simulink model "gm_test_cost_function_only_without_delays"  (R2022a)
settings: Solver=FixedStepDiscrete  StartTime=0.0  StopTime=10.0  RelTol=1e-3
undefined symbols (not defined in the file or in its folder): f_c
libraries: hdlmdlgenlib x64
(part 1 of 2)
settings Model: Creator=Andre Merx  LastModifiedBy=Andre Merx
settings SolverCC: AlgebraicLoopSolver=TrustRegion
settings DataIOCC: LimitDataPoints=on  SaveOutput=off  SaveTime=off
settings OptimizationCC: BlockReduction=off  ConditionallyExecuteInputs=off  DefaultParameterBehavior=Inlined  LifeSpan=inf
settings DebuggingCC: AlgebraicLoopMsg=error  InheritedTsInSrcMsg=none  SingleTaskRateTransMsg=error  UnconnectedInputMsg=warning  UnconnectedOutputMsg=warning  UnconnectedLineMsg=warning  AllowSymbolicDim=off  StrictBusMsg=ErrorOnBusTreatedAsVector  SFUnexpectedBacktrackingDiag=warning  SFNoUnconditionalDefaultTransitionDiag=warning  SFExecutionAtInitializationDiag=none  SFMachineParentedDataDiag=warning  ArithmeticOperatorsInVariantConditions=warning
settings HardwareCC: ProdBitPerPointer=32  ProdBitPerSizeT=32  ProdBitPerPtrDiffT=32  ProdLargestAtomicFloat=None  ProdIntDivRoundTo=Undefined  ProdEndianess=Unspecified  ProdWordSize=32  ProdHWDeviceType=ASIC/FPGA->ASIC/FPGA  ProdEqTarget=off
settings SFSimCC: SimUseLocalCustomCode=off  CustomCodeUndefinedFunction=UseInterfaceOnly
settings RTWCC: RTWUseLocalCustomCode=off
settings CodeAppCC: StateflowObjectComments=on
settings GRTTargetCC: TargetLangStandard=C89/C90 (ANSI)
settings ConfigComp: CovScope=ReferencedModels  CovMetricSettings=dw  CovSaveCumulativeToWorkspaceVar=on  CovSaveSingleToWorkspaceVar=on  CovExternalEMLEnable=off  CovSFcnEnable=off

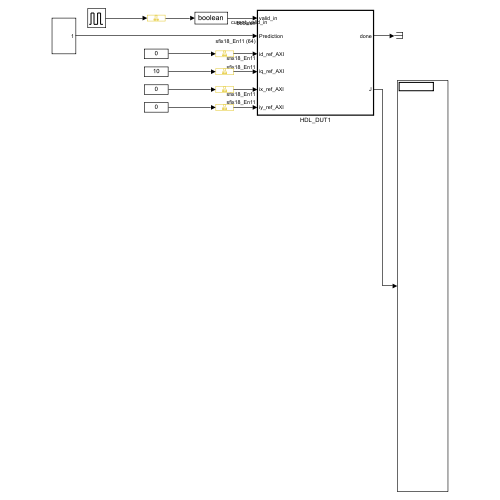
[thumbnail: Simulink's stored preview of the top-level diagram]
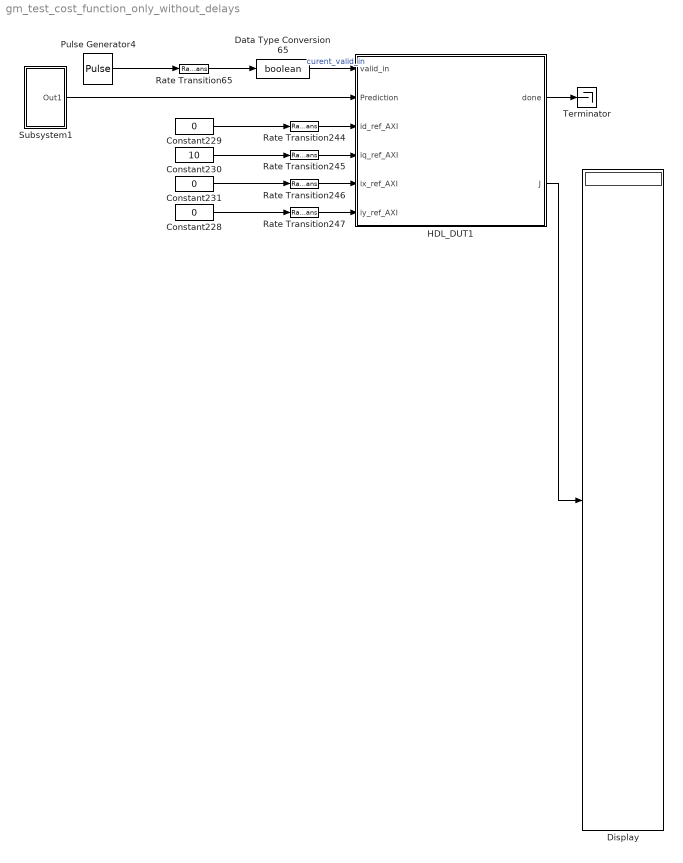
== system gm_test_cost_function_only_without_delays ==
  Constant228 : Constant  Value=0  OutDataTypeStr=fixdt(1,18,11)  SampleTime=-1
  Constant229 : Constant  Value=0  OutDataTypeStr=fixdt(1,18,11)  SampleTime=-1
  Constant230 : Constant  Value=10  OutDataTypeStr=fixdt(1,18,11)  SampleTime=-1
  Constant231 : Constant  Value=0  OutDataTypeStr=fixdt(1,18,11)  SampleTime=-1
  Data Type Conversion65 : DataTypeConversion  OutDataTypeStr=boolean  SaturateOnIntegerOverflow=off  RndMeth=Floor
  Display : Display
  HDL_DUT1 : Subsystem  TreatAsAtomicUnit=on
  Pulse Generator4 : DiscretePulseGenerator  PulseType=Time based  Period=1/f_c
  Rate Transition{65,244..247} (5 alike) : RateTransition  OutPortSampleTime=Rt
  Subsystem1 : Subsystem
  Terminator : Terminator
  wires:
  HDL_DUT1/2(J) -> Display/1
  HDL_DUT1/1(done) -> Terminator/1
  Data Type Conversion65/1 -> HDL_DUT1/1(valid_in)  "curent_valid_in"
  Rate Transition65/1 -> Data Type Conversion65/1
  Pulse Generator4/1 -> Rate Transition65/1
  Rate Transition244/1 -> HDL_DUT1/3(id_ref_AXI)
  Rate Transition246/1 -> HDL_DUT1/5(ix_ref_AXI)
  Constant230/1 -> Rate Transition245/1
  Constant229/1 -> Rate Transition244/1
  Subsystem1/1(Out1) -> HDL_DUT1/2(Prediction)
  Rate Transition245/1 -> HDL_DUT1/4(iq_ref_AXI)
  Rate Transition247/1 -> HDL_DUT1/6(iy_ref_AXI)
  Constant231/1 -> Rate Transition246/1
  Constant228/1 -> Rate Transition247/1

== system gm_test_cost_function_only_without_delays/HDL_DUT1 ==
  valid_in : Inport  OutDataTypeStr=boolean  PortDimensions=1  SampleTime=1e-08
  Prediction : Inport  Port=2  OutDataTypeStr=fixdt(1, 18, 11)  PortDimensions=[64]  SampleTime=1e-08
  id_ref_AXI : Inport  Port=3  OutDataTypeStr=fixdt(1, 18, 11)  PortDimensions=1  SampleTime=1e-08
  iq_ref_AXI : Inport  Port=4  OutDataTypeStr=fixdt(1, 18, 11)  PortDimensions=1  SampleTime=1e-08
  ix_ref_AXI : Inport  Port=5  OutDataTypeStr=fixdt(1, 18, 11)  PortDimensions=1  SampleTime=1e-08
  iy_ref_AXI : Inport  Port=6  OutDataTypeStr=fixdt(1, 18, 11)  PortDimensions=1  SampleTime=1e-08
  Delay{7..10,33} (5 alike) : Delay  DelayLength=double(1)  InitialCondition=0  SampleTime=1e-08
  Detect Rise Positive : Subsystem  mask(Detect Rise Positive){vinit=double(0), InputProcessing=Elements as channels (sample based), OutDataTypeStr=boolean}
      mask prompts: vinit "Simulink:masks:InitialCondition_MP"; InputProcessing "Simulink:masks:InputProcessing_MP"; OutDataTypeStr "Simulink:masks:OutputDataType_MP"
      mask help: Simulink:masks:DetectRisePositive_MD
      mask init:
      | InputProcessing = 'Elements as channels (sample based)';
      | OutDataTypeStr = 'boolean';
      | vinit = double(0);
      mask TypeOptions InputProcessing: Simulink:masks:ColumnsAsChannelsFrameBased | Simulink:masks:ElementsAsChannelsSampleBased
      mask TypeOptions OutDataTypeStr: Simulink:masks:uint8 | Simulink:masks:boolean
      mask Display: fprintf('U > 0\n&  NOT\nU/z > 0')
  Subsystem : Subsystem
  Switch_on{1..4,14} (5 alike) : Switch  Threshold=double(1)  OutDataTypeStr=fixdt(1, 18, 11)  RndMeth=Simplest  SampleTime=1e-08  SaturateOnIntegerOverflow=off  InputSameDT=off
  mux : Mux  Inputs=16
  done : Outport  SampleTime=1e-08
  J : Outport  Port=2  SampleTime=1e-08
  wires:
  valid_in/1 -> Detect Rise Positive/1(U)
  Prediction/1 -> Switch_on4/1
  id_ref_AXI/1 -> Switch_on3/1
  iq_ref_AXI/1 -> Switch_on2/1
  ix_ref_AXI/1 -> Switch_on1/1
  iy_ref_AXI/1 -> Switch_on14/1
  Delay10/1 -> Switch_on4/3
  Delay33/1 -> Switch_on14/3
  Delay7/1 -> Switch_on1/3
  Delay8/1 -> Switch_on2/3
  Delay9/1 -> Switch_on3/3
  Detect Rise Positive/1(Y) -> Switch_on4/2, Switch_on3/2, Switch_on2/2, Switch_on14/2, Switch_on1/2, done/1
  mux/1 -> J/1
  Subsystem/1(J1) -> mux/1
  Subsystem/2(J2) -> mux/2
  Subsystem/3(J3) -> mux/3
  Subsystem/4(J4) -> mux/4
  Subsystem/5(J5) -> mux/5
  Subsystem/6(J6) -> mux/6
  Subsystem/7(J7) -> mux/7
  Subsystem/8(J8) -> mux/8
  Subsystem/9(J9) -> mux/9
  Subsystem/10(J10) -> mux/10
  Subsystem/11(J11) -> mux/11
  Subsystem/12(J12) -> mux/12
  Subsystem/13(J13) -> mux/13
  Subsystem/14(J14) -> mux/14
  Subsystem/15(J15) -> mux/15
  Subsystem/16(J16) -> mux/16
  Switch_on1/1 -> Delay7/1, Subsystem/4(ix_ref)
  Switch_on14/1 -> Delay33/1, Subsystem/5(iy_ref)
  Switch_on2/1 -> Delay8/1, Subsystem/3(iq_ref)
  Switch_on3/1 -> Delay9/1, Subsystem/2(id_ref)
  Switch_on4/1 -> Delay10/1, Subsystem/1(Predicton)

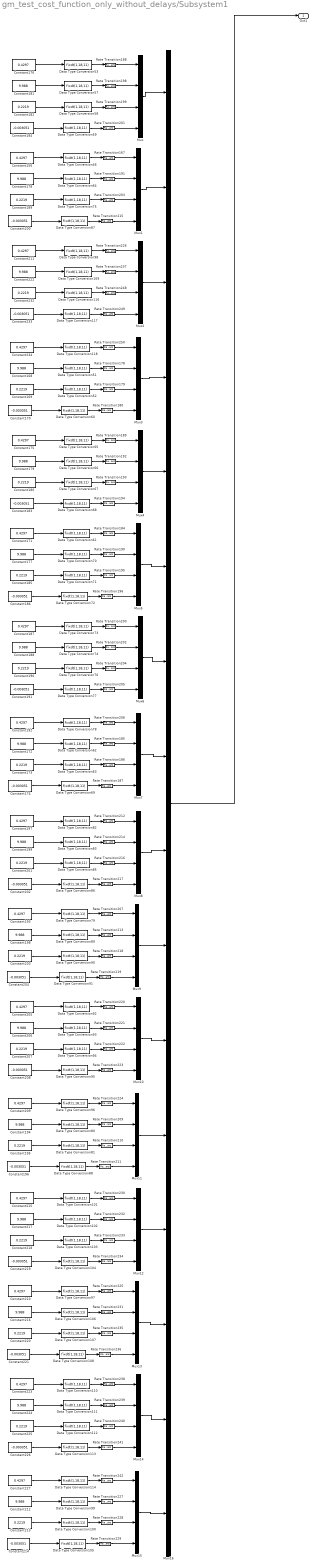
== system gm_test_cost_function_only_without_delays/Subsystem1 ==
  Constant{156,171,175..176,187,192..193,197,205,209..211,215,223,227,234} (16 alike) : Constant  Value=0.4297
  Constant{168,172,177..179,181,188,194,198..199,206,212,216..217,222,224} (16 alike) : Constant  Value=9.988
  Constant{169,173,180,182,185,189..190,195,201,203,207,213,218,220,225,232} (16 alike) : Constant  Value=0.2219
  Constant{170,174,183..184,186,191,196,200,202,204,208,214,219,221,226,233} (16 alike) : Constant  Value=-0.003051
  Data Type Conversion{46,51..53,57..83,85..114,116..118} (64 alike) : DataTypeConversion  OutDataTypeStr=fixdt(1,18,11)  SaturateOnIntegerOverflow=off  RndMeth=Floor
  Mux{,1..15} (16 alike) : Mux
  Mux16 : Mux  Inputs=16
  Rate Transition{167,178..180,184..196,198..207,209..242,248..250} (64 alike) : RateTransition  OutPortSampleTime=Rt
  Out1 : Outport
  wires:
  Data Type Conversion90/1 -> Rate Transition218/1
  Rate Transition223/1 -> Mux10/4
  Data Type Conversion92/1 -> Rate Transition220/1
  Constant197/1 -> Data Type Conversion82/1
  Rate Transition214/1 -> Mux8/2
  Rate Transition206/1 -> Mux7/1
  Data Type Conversion95/1 -> Rate Transition223/1
  Constant207/1 -> Data Type Conversion94/1
  Rate Transition221/1 -> Mux10/2
  Data Type Conversion51/1 -> Rate Transition178/1
  Data Type Conversion89/1 -> Rate Transition213/1
  Rate Transition185/1 -> Mux7/2
  Data Type Conversion81/1 -> Rate Transition210/1
  Constant189/1 -> Data Type Conversion75/1
  Rate Transition191/1 -> Mux1/2
  Rate Transition233/1 -> Mux12/3
  Data Type Conversion76/1 -> Rate Transition204/1
  Constant203/1 -> Data Type Conversion90/1
  Data Type Conversion96/1 -> Rate Transition224/1
  Rate Transition213/1 -> Mux9/2
  Constant198/1 -> Data Type Conversion89/1
  Constant218/1 -> Data Type Conversion103/1
  Data Type Conversion94/1 -> Rate Transition222/1
  Data Type Conversion91/1 -> Rate Transition219/1
  Data Type Conversion110/1 -> Rate Transition238/1
  Data Type Conversion103/1 -> Rate Transition233/1
  Rate Transition212/1 -> Mux8/1
  Rate Transition216/1 -> Mux8/3
  Constant191/1 -> Data Type Conversion77/1
  Data Type Conversion58/1 -> Rate Transition199/1
  Rate Transition204/1 -> Mux6/3
  Data Type Conversion113/1 -> Rate Transition241/1
  Constant226/1 -> Data Type Conversion113/1
  Constant192/1 -> Data Type Conversion78/1
  Constant217/1 -> Data Type Conversion102/1
  Data Type Conversion98/1 -> Rate Transition226/1
  Rate Transition219/1 -> Mux9/4
  Mux4/1 -> Mux16/5
  Constant171/1 -> Data Type Conversion61/1
  Constant234/1 -> Data Type Conversion118/1
  Data Type Conversion106/1 -> Rate Transition231/1
  Rate Transition225/1 -> Mux13/1
  Rate Transition207/1 -> Mux9/1
  Rate Transition234/1 -> Mux12/4
  Rate Transition229/1 -> Mux15/4
  Rate Transition240/1 -> Mux14/3
  Constant213/1 -> Data Type Conversion100/1
  Constant216/1 -> Data Type Conversion106/1
  Data Type Conversion99/1 -> Rate Transition227/1
  Rate Transition231/1 -> Mux13/2
  Rate Transition241/1 -> Mux14/4
  Mux3/1 -> Mux16/4
  Rate Transition239/1 -> Mux14/2
  Rate Transition218/1 -> Mux9/3
  Mux2/1 -> Mux16/3
  Mux9/1 -> Mux16/10
  Rate Transition228/1 -> Mux15/3
  Data Type Conversion105/1 -> Rate Transition229/1
  Mux5/1 -> Mux16/6
  Data Type Conversion97/1 -> Rate Transition225/1
  Mux1/1 -> Mux16/2
  Rate Transition209/1 -> Mux11/2
  Data Type Conversion77/1 -> Rate Transition205/1
  Constant219/1 -> Data Type Conversion104/1
  Constant204/1 -> Data Type Conversion91/1
  Constant212/1 -> Data Type Conversion99/1
  Mux6/1 -> Mux16/7
  Data Type Conversion52/1 -> Rate Transition179/1
  Rate Transition205/1 -> Mux6/4
  Data Type Conversion46/1 -> Rate Transition167/1
  Constant200/1 -> Data Type Conversion87/1
  Data Type Conversion68/1 -> Rate Transition194/1
  Data Type Conversion104/1 -> Rate Transition234/1
  Data Type Conversion85/1 -> Rate Transition216/1
  Mux11/1 -> Mux16/12
  Mux12/1 -> Mux16/13
  Constant227/1 -> Data Type Conversion114/1
  Rate Transition220/1 -> Mux10/1
  Data Type Conversion111/1 -> Rate Transition239/1
  Data Type Conversion82/1 -> Rate Transition212/1
  Rate Transition179/1 -> Mux3/3
  Mux14/1 -> Mux16/15
  Rate Transition242/1 -> Mux15/1
  Rate Transition236/1 -> Mux13/4
  Rate Transition249/1 -> Mux2/4
  Data Type Conversion107/1 -> Rate Transition235/1
  Constant224/1 -> Data Type Conversion111/1
  Constant210/1 -> Data Type Conversion97/1
  Data Type Conversion62/1 -> Rate Transition185/1
  Constant186/1 -> Data Type Conversion72/1
  Data Type Conversion112/1 -> Rate Transition240/1
  Rate Transition195/1 -> Mux5/3
  Data Type Conversion78/1 -> Rate Transition206/1
  Constant206/1 -> Data Type Conversion93/1
  Constant190/1 -> Data Type Conversion76/1
  Rate Transition180/1 -> Mux3/4
  Constant223/1 -> Data Type Conversion110/1
  Rate Transition198/1 -> Mux/2
  Data Type Conversion59/1 -> Rate Transition201/1
  Constant194/1 -> Data Type Conversion80/1
  Constant185/1 -> Data Type Conversion71/1
  Constant225/1 -> Data Type Conversion112/1
  Rate Transition235/1 -> Mux13/3
  Constant174/1 -> Data Type Conversion69/1
  Data Type Conversion109/1 -> Rate Transition237/1
  Data Type Conversion114/1 -> Rate Transition242/1
  Constant177/1 -> Data Type Conversion70/1
  Rate Transition203/1 -> Mux1/3
  Mux10/1 -> Mux16/11
  Constant173/1 -> Data Type Conversion63/1
  Constant201/1 -> Data Type Conversion85/1
  Constant178/1 -> Data Type Conversion64/1
  Data Type Conversion60/1 -> Rate Transition180/1
  Data Type Conversion73/1 -> Rate Transition200/1
  Data Type Conversion101/1 -> Rate Transition230/1
  Rate Transition248/1 -> Mux2/3
  Constant181/1 -> Data Type Conversion57/1
  Constant156/1 -> Data Type Conversion46/1
  Rate Transition237/1 -> Mux2/2
  Data Type Conversion57/1 -> Rate Transition198/1
  Rate Transition211/1 -> Mux11/4
  Rate Transition226/1 -> Mux2/1
  Mux15/1 -> Mux16/16
  Constant232/1 -> Data Type Conversion116/1
  Constant209/1 -> Data Type Conversion96/1
  Rate Transition188/1 -> Mux/1
  Rate Transition186/1 -> Mux7/3
  Rate Transition199/1 -> Mux/3
  Data Type Conversion67/1 -> Rate Transition193/1
  Constant211/1 -> Data Type Conversion98/1
  Constant196/1 -> Data Type Conversion88/1
  Rate Transition167/1 -> Mux1/1
  Constant233/1 -> Data Type Conversion117/1
  Data Type Conversion100/1 -> Rate Transition228/1
  Rate Transition217/1 -> Mux8/4
  Constant180/1 -> Data Type Conversion67/1
  Rate Transition194/1 -> Mux4/4
  Data Type Conversion53/1 -> Rate Transition188/1
  Constant215/1 -> Data Type Conversion101/1
  Data Type Conversion80/1 -> Rate Transition209/1
  Data Type Conversion118/1 -> Rate Transition250/1
  Mux16/1 -> Out1/1
  Constant221/1 -> Data Type Conversion108/1
  Constant179/1 -> Data Type Conversion66/1
  Constant184/1 -> Data Type Conversion59/1
  Constant222/1 -> Data Type Conversion109/1
  Data Type Conversion102/1 -> Rate Transition232/1
  Rate Transition250/1 -> Mux3/1
  Rate Transition230/1 -> Mux12/1
  Rate Transition200/1 -> Mux6/1
  Constant176/1 -> Data Type Conversion53/1
  Mux8/1 -> Mux16/9
  Data Type Conversion116/1 -> Rate Transition248/1
  Rate Transition238/1 -> Mux14/1
  Data Type Conversion86/1 -> Rate Transition217/1
  Constant170/1 -> Data Type Conversion60/1
  Constant208/1 -> Data Type Conversion95/1
  Data Type Conversion108/1 -> Rate Transition236/1
  Rate Transition210/1 -> Mux11/3
  Rate Transition192/1 -> Mux4/2
  Data Type Conversion74/1 -> Rate Transition202/1
  Constant199/1 -> Data Type Conversion83/1
  Constant187/1 -> Data Type Conversion73/1
  Rate Transition227/1 -> Mux15/2
  Data Type Conversion64/1 -> Rate Transition191/1
  Data Type Conversion93/1 -> Rate Transition221/1
  Data Type Conversion61/1 -> Rate Transition184/1
  Constant202/1 -> Data Type Conversion86/1
  Rate Transition232/1 -> Mux12/2
  Constant172/1 -> Data Type Conversion62/1
  Rate Transition224/1 -> Mux11/1
  Mux/1 -> Mux16/1
  Constant214/1 -> Data Type Conversion105/1
  Constant195/1 -> Data Type Conversion81/1
  Rate Transition189/1 -> Mux4/1
  Constant188/1 -> Data Type Conversion74/1
  Rate Transition222/1 -> Mux10/3
  Rate Transition187/1 -> Mux7/4
  Constant183/1 -> Data Type Conversion68/1
  Constant168/1 -> Data Type Conversion51/1
  Rate Transition196/1 -> Mux5/4
  Rate Transition190/1 -> Mux5/2
  Data Type Conversion66/1 -> Rate Transition192/1
  Data Type Conversion65/1 -> Rate Transition189/1
  Data Type Conversion79/1 -> Rate Transition207/1
  Rate Transition184/1 -> Mux5/1
  Mux7/1 -> Mux16/8
  Rate Transition201/1 -> Mux/4
  Data Type Conversion75/1 -> Rate Transition203/1
  Data Type Conversion83/1 -> Rate Transition214/1
  Data Type Conversion72/1 -> Rate Transition196/1
  Data Type Conversion63/1 -> Rate Transition186/1
  Rate Transition193/1 -> Mux4/3
  Constant175/1 -> Data Type Conversion65/1
  Rate Transition178/1 -> Mux3/2
  Constant169/1 -> Data Type Conversion52/1
  Data Type Conversion70/1 -> Rate Transition190/1
  Rate Transition202/1 -> Mux6/2
  Data Type Conversion88/1 -> Rate Transition211/1
  Mux13/1 -> Mux16/14
  Constant182/1 -> Data Type Conversion58/1
  Constant193/1 -> Data Type Conversion79/1
  Data Type Conversion87/1 -> Rate Transition215/1
  Data Type Conversion117/1 -> Rate Transition249/1
  Data Type Conversion71/1 -> Rate Transition195/1
  Data Type Conversion69/1 -> Rate Transition187/1
  Rate Transition215/1 -> Mux1/4
  Constant205/1 -> Data Type Conversion92/1
  Constant220/1 -> Data Type Conversion107/1

== system gm_test_cost_function_only_without_delays/HDL_DUT1/Detect Rise Positive ==
  note: Edge
  note: U(k)
  U : Inport  OutDataTypeStr=boolean  SampleTime=1e-08
  Delay Input1 : UnitDelay  Description=Store in Global RAM  DisableCoverage=on  InitialCondition=vinit  SampleTime=-1  HasFrameUpgradeWarning=on
  FixPt Relational Operator : RelationalOperator  Operator=>  OutDataTypeStr=boolean  ZeroCross=off  InputSameDT=off
  Positive : Subsystem  mask(Compare To Zero){relop=>, OutDataTypeStr=boolean, ZeroCross=off}
      mask prompts: relop "Simulink:masks:Operator_MP"; OutDataTypeStr "Simulink:masks:OutputDataType_MP"; ZeroCross "Simulink:masks:EnableZerocrossingDetection_MP"
      mask help: Simulink:masks:CompareToZero_MD
      mask init:
      | OutDataTypeStr = 'boolean';
      | ZeroCross = 'off';
      | blkName = 'test_cost_function_only_without_delays/HDL_DUT1/Detect Rise\nPositive/Positive';
      | relop = '>';
      | setValue = 'boolean';
      mask TypeOptions relop: == | ~= | < | <= | >= | >
      mask TypeOptions OutDataTypeStr: Simulink:masks:uint8 | Simulink:masks:boolean
      mask Callback ZeroCross: sl('zeroCrossEnable', gcbh);
      mask Display: disp([relop,' 0'])
  Y : Outport  SampleTime=1e-08
  wires:
  U/1 -> Positive/1(u)
  Delay Input1/1 -> FixPt Relational Operator/2
  FixPt Relational Operator/1 -> Y/1
  Positive/1(y) -> FixPt Relational Operator/1, Delay Input1/1

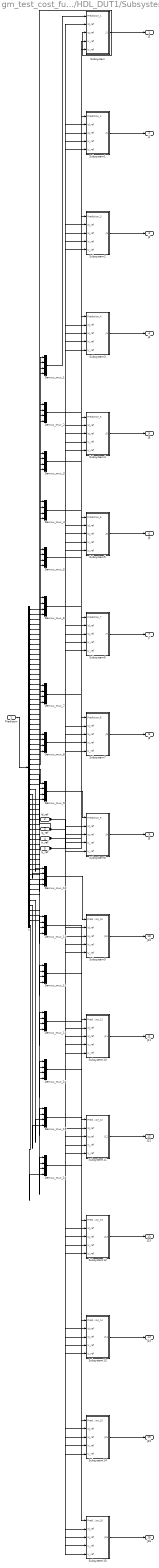
== system gm_test_cost_function_only_without_delays/HDL_DUT1/Subsystem ==
  Predicton : Inport  OutDataTypeStr=fixdt(1, 18, 11)  PortDimensions=[64]  SampleTime=1e-08
  id_ref : Inport  Port=2  OutDataTypeStr=fixdt(1, 18, 11)  PortDimensions=1  SampleTime=1e-08
  iq_ref : Inport  Port=3  OutDataTypeStr=fixdt(1, 18, 11)  PortDimensions=1  SampleTime=1e-08
  ix_ref : Inport  Port=4  OutDataTypeStr=fixdt(1, 18, 11)  PortDimensions=1  SampleTime=1e-08
  iy_ref : Inport  Port=5  OutDataTypeStr=fixdt(1, 18, 11)  PortDimensions=1  SampleTime=1e-08
  Demux_mux_{1..16} (16 alike) : Mux
  Subsystem : Subsystem
  Subsystem1 : Subsystem
  Subsystem10 : Subsystem
  Subsystem11 : Subsystem
  Subsystem12 : Subsystem
  Subsystem13 : Subsystem
  Subsystem14 : Subsystem
  Subsystem15 : Subsystem
  Subsystem2 : Subsystem
  Subsystem3 : Subsystem
  Subsystem4 : Subsystem
  Subsystem5 : Subsystem
  Subsystem6 : Subsystem
  Subsystem7 : Subsystem
  Subsystem8 : Subsystem
  Subsystem9 : Subsystem
  t : Demux  Outputs=64
  J1 : Outport  SampleTime=1e-08
  J2 : Outport  Port=2  SampleTime=1e-08
  J3 : Outport  Port=3  SampleTime=1e-08
  J4 : Outport  Port=4  SampleTime=1e-08
  J5 : Outport  Port=5  SampleTime=1e-08
  J6 : Outport  Port=6  SampleTime=1e-08
  J7 : Outport  Port=7  SampleTime=1e-08
  J8 : Outport  Port=8  SampleTime=1e-08
  J9 : Outport  Port=9  SampleTime=1e-08
  J10 : Outport  Port=10  SampleTime=1e-08
  J11 : Outport  Port=11  SampleTime=1e-08
  J12 : Outport  Port=12  SampleTime=1e-08
  J13 : Outport  Port=13  SampleTime=1e-08
  J14 : Outport  Port=14  SampleTime=1e-08
  J15 : Outport  Port=15  SampleTime=1e-08
  J16 : Outport  Port=16  SampleTime=1e-08
  wires:
  Predicton/1 -> t/1
  id_ref/1 -> Subsystem15/2(id_ref), Subsystem14/2(id_ref), Subsystem13/2(id_ref), Subsystem12/2(id_ref), Subsystem11/2(id_ref), Subsystem10/2(id_ref), Subsystem9/2(id_ref), Subsystem8/2(id_ref), Subsystem7/2(id_ref), Subsystem6/2(id_ref), Subsystem5/2(id_ref), Subsystem4/2(id_ref), Subsystem3/2(id_ref), Subsystem2/2(id_ref), Subsystem1/2(id_ref), Subsystem/2(id_ref)
  iq_ref/1 -> Subsystem/3(iq_ref), Subsystem15/3(iq_ref), Subsystem14/3(iq_ref), Subsystem13/3(iq_ref), Subsystem12/3(iq_ref), Subsystem11/3(iq_ref), Subsystem10/3(iq_ref), Subsystem9/3(iq_ref), Subsystem8/3(iq_ref), Subsystem7/3(iq_ref), Subsystem6/3(iq_ref), Subsystem5/3(iq_ref), Subsystem4/3(iq_ref), Subsystem3/3(iq_ref), Subsystem2/3(iq_ref), Subsystem1/3(iq_ref)
  ix_ref/1 -> Subsystem/4(ix_ref), Subsystem15/4(ix_ref), Subsystem14/4(ix_ref), Subsystem13/4(ix_ref), Subsystem12/4(ix_ref), Subsystem11/4(ix_ref), Subsystem10/4(ix_ref), Subsystem9/4(ix_ref), Subsystem8/4(ix_ref), Subsystem7/4(ix_ref), Subsystem6/4(ix_ref), Subsystem5/4(ix_ref), Subsystem4/4(ix_ref), Subsystem3/4(ix_ref), Subsystem2/4(ix_ref), Subsystem1/4(ix_ref)
  iy_ref/1 -> Subsystem/5(iy_ref), Subsystem15/5(iy_ref), Subsystem14/5(iy_ref), Subsystem13/5(iy_ref), Subsystem12/5(iy_ref), Subsystem11/5(iy_ref), Subsystem10/5(iy_ref), Subsystem9/5(iy_ref), Subsystem8/5(iy_ref), Subsystem7/5(iy_ref), Subsystem6/5(iy_ref), Subsystem5/5(iy_ref), Subsystem4/5(iy_ref), Subsystem3/5(iy_ref), Subsystem2/5(iy_ref), Subsystem1/5(iy_ref)
  Demux_mux_1/1 -> Subsystem/1(Prediction_1)
  Demux_mux_2/1 -> Subsystem1/1(Prediction_2)
  Demux_mux_3/1 -> Subsystem2/1(Prediction_3)
  Demux_mux_4/1 -> Subsystem3/1(Prediction_4)
  Demux_mux_5/1 -> Subsystem4/1(Prediction_5)
  Demux_mux_6/1 -> Subsystem5/1(Prediction_6)
  Demux_mux_7/1 -> Subsystem6/1(Prediction_7)
  Demux_mux_8/1 -> Subsystem7/1(Prediction_8)
  Demux_mux_9/1 -> Subsystem8/1(Prediction_9)
  Demux_mux_10/1 -> Subsystem9/1(Prediction_10)
  Demux_mux_11/1 -> Subsystem10/1(Prediction_11)
  Demux_mux_12/1 -> Subsystem11/1(Prediction_12)
  Demux_mux_13/1 -> Subsystem12/1(Prediction_13)
  Demux_mux_14/1 -> Subsystem13/1(Prediction_14)
  Demux_mux_15/1 -> Subsystem14/1(Prediction_15)
  Demux_mux_16/1 -> Subsystem15/1(Prediction_16)
  Subsystem/1(J1) -> J1/1
  Subsystem1/1(J2) -> J2/1
  Subsystem10/1(J11) -> J11/1
  Subsystem11/1(J12) -> J12/1
  Subsystem12/1(J13) -> J13/1
  Subsystem13/1(J14) -> J14/1
  Subsystem14/1(J15) -> J15/1
  Subsystem15/1(J16) -> J16/1
  Subsystem2/1(J3) -> J3/1
  Subsystem3/1(J4) -> J4/1
  Subsystem4/1(J5) -> J5/1
  Subsystem5/1(J6) -> J6/1
  Subsystem6/1(J7) -> J7/1
  Subsystem7/1(J8) -> J8/1
  Subsystem8/1(J9) -> J9/1
  Subsystem9/1(J10) -> J10/1
  t/1 -> Demux_mux_1/1
  t/2 -> Demux_mux_1/2
  t/3 -> Demux_mux_1/3
  t/4 -> Demux_mux_1/4
  t/5 -> Demux_mux_2/1
  t/6 -> Demux_mux_2/2
  t/7 -> Demux_mux_2/3
  t/8 -> Demux_mux_2/4
  t/9 -> Demux_mux_3/1
  t/10 -> Demux_mux_3/2
  t/11 -> Demux_mux_3/3
  t/12 -> Demux_mux_3/4
  t/13 -> Demux_mux_4/1
  t/14 -> Demux_mux_4/2
  t/15 -> Demux_mux_4/3
  t/16 -> Demux_mux_4/4
  t/17 -> Demux_mux_5/1
  t/18 -> Demux_mux_5/2
  t/19 -> Demux_mux_5/3
  t/20 -> Demux_mux_5/4
  t/21 -> Demux_mux_6/1
  t/22 -> Demux_mux_6/2
  t/23 -> Demux_mux_6/3
  t/24 -> Demux_mux_6/4
  t/25 -> Demux_mux_7/1
  t/26 -> Demux_mux_7/2
  t/27 -> Demux_mux_7/3
  t/28 -> Demux_mux_7/4
  t/29 -> Demux_mux_8/1
  t/30 -> Demux_mux_8/2
  t/31 -> Demux_mux_8/3
  t/32 -> Demux_mux_8/4
  t/33 -> Demux_mux_9/1
  t/34 -> Demux_mux_9/2
  t/35 -> Demux_mux_9/3
  t/36 -> Demux_mux_9/4
  t/37 -> Demux_mux_10/1
  t/38 -> Demux_mux_10/2
  t/39 -> Demux_mux_10/3
  t/40 -> Demux_mux_10/4
  t/41 -> Demux_mux_11/1
  t/42 -> Demux_mux_11/2
  t/43 -> Demux_mux_11/3
  t/44 -> Demux_mux_11/4
  t/45 -> Demux_mux_12/1
  t/46 -> Demux_mux_12/2
  t/47 -> Demux_mux_12/3
  t/48 -> Demux_mux_12/4
  t/49 -> Demux_mux_13/1
  t/50 -> Demux_mux_13/2
  t/51 -> Demux_mux_13/3
  t/52 -> Demux_mux_13/4
  t/53 -> Demux_mux_14/1
  t/54 -> Demux_mux_14/2
  t/55 -> Demux_mux_14/3
  t/56 -> Demux_mux_14/4
  t/57 -> Demux_mux_15/1
  t/58 -> Demux_mux_15/2
  t/59 -> Demux_mux_15/3
  t/60 -> Demux_mux_15/4
  t/61 -> Demux_mux_16/1
  t/62 -> Demux_mux_16/2
  t/63 -> Demux_mux_16/3
  t/64 -> Demux_mux_16/4

== system gm_test_cost_function_only_without_delays/HDL_DUT1/Detect Rise Positive/Positive ==
  u : Inport  OutDataTypeStr=boolean  SampleTime=1e-08
  Compare : RelationalOperator  Operator=>  OutDataTypeStr=boolean  ZeroCross=off
  Constant : Constant  DisableCoverage=on  Value=0  OutDataTypeStr=Inherit: Inherit via back propagation  SampleTime=-1  PreserveConstantTs=on
  y : Outport  SampleTime=1e-08
  wires:
  u/1 -> Compare/1
  Compare/1 -> y/1
  Constant/1 -> Compare/2

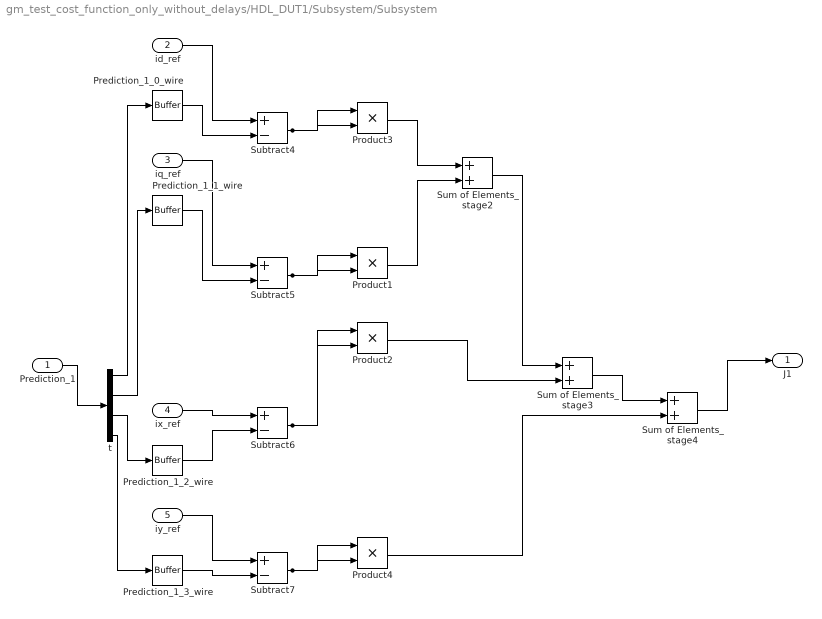
== system gm_test_cost_function_only_without_delays/HDL_DUT1/Subsystem/Subsystem ==
  Prediction_1 : Inport  OutDataTypeStr=fixdt(1, 18, 11)  PortDimensions=[4]  SampleTime=1e-08
  id_ref : Inport  Port=2  OutDataTypeStr=fixdt(1, 18, 11)  PortDimensions=1  SampleTime=1e-08
  iq_ref : Inport  Port=3  OutDataTypeStr=fixdt(1, 18, 11)  PortDimensions=1  SampleTime=1e-08
  ix_ref : Inport  Port=4  OutDataTypeStr=fixdt(1, 18, 11)  PortDimensions=1  SampleTime=1e-08
  iy_ref : Inport  Port=5  OutDataTypeStr=fixdt(1, 18, 11)  PortDimensions=1  SampleTime=1e-08
  Prediction_1_0_wire : hdlmdlgenlib/Buffer
      settings: SourceProductBaseCode=SL
  Prediction_1_1_wire : hdlmdlgenlib/Buffer
      settings: SourceProductBaseCode=SL
  Prediction_1_2_wire : hdlmdlgenlib/Buffer
      settings: SourceProductBaseCode=SL
  Prediction_1_3_wire : hdlmdlgenlib/Buffer
      settings: SourceProductBaseCode=SL
  Product{1..4} (4 alike) : Product  Inputs=**  OutDataTypeStr=fixdt(1, 20, 11)  SampleTime=1e-08
  Subtract{4..7} (4 alike) : Sum  Inputs=+-  AccumDataTypeStr=fixdt(1, 19, 11)  OutDataTypeStr=fixdt(1, 20, 11)  SampleTime=1e-08
  Sum of Elements_stage2 : Sum  AccumDataTypeStr=fixdt(1, 22, 11)  OutDataTypeStr=fixdt(1, 21, 11)  SampleTime=1e-08
  Sum of Elements_stage3 : Sum  AccumDataTypeStr=fixdt(1, 22, 11)  OutDataTypeStr=fixdt(1, 22, 11)  SampleTime=1e-08
  Sum of Elements_stage4 : Sum  AccumDataTypeStr=fixdt(1, 22, 11)  OutDataTypeStr=fixdt(1, 20, 11)  SampleTime=1e-08
  t : Demux
  J1 : Outport  SampleTime=1e-08
  wires:
  Prediction_1/1 -> t/1
  id_ref/1 -> Subtract4/1
  iq_ref/1 -> Subtract5/1
  ix_ref/1 -> Subtract6/1
  iy_ref/1 -> Subtract7/1
  Prediction_1_0_wire/1 -> Subtract4/2
  Prediction_1_1_wire/1 -> Subtract5/2
  Prediction_1_2_wire/1 -> Subtract6/2
  Prediction_1_3_wire/1 -> Subtract7/2
  Product1/1 -> Sum of Elements_stage2/2
  Product2/1 -> Sum of Elements_stage3/2
  Product3/1 -> Sum of Elements_stage2/1
  Product4/1 -> Sum of Elements_stage4/2
  Subtract4/1 -> Product3/2, Product3/1
  Subtract5/1 -> Product1/2, Product1/1
  Subtract6/1 -> Product2/2, Product2/1
  Subtract7/1 -> Product4/2, Product4/1
  Sum of Elements_stage4/1 -> J1/1
  t/1 -> Prediction_1_0_wire/1
  t/2 -> Prediction_1_1_wire/1
  t/3 -> Prediction_1_2_wire/1
  t/4 -> Prediction_1_3_wire/1
  Sum of Elements_stage2/1 -> Sum of Elements_stage3/1
  Sum of Elements_stage3/1 -> Sum of Elements_stage4/1

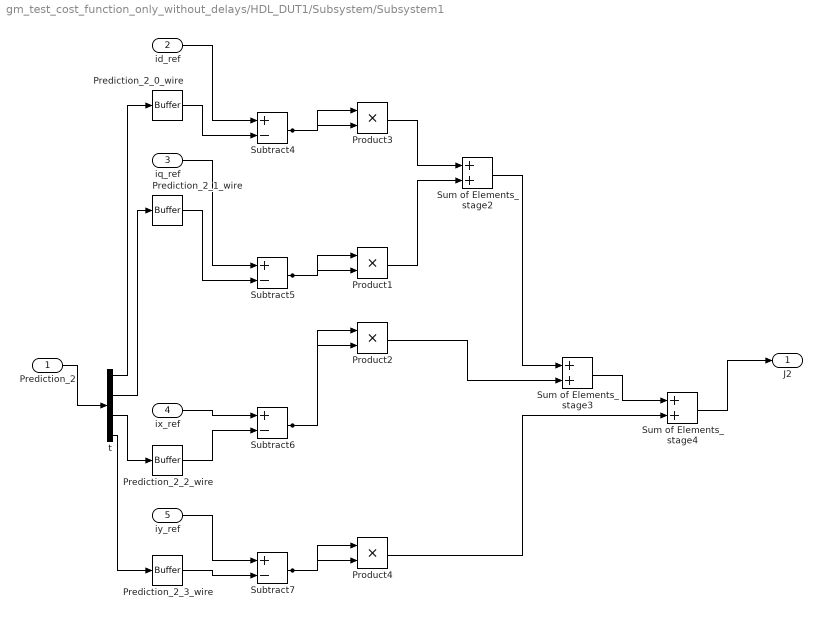
== system gm_test_cost_function_only_without_delays/HDL_DUT1/Subsystem/Subsystem1 ==
  Prediction_2 : Inport  OutDataTypeStr=fixdt(1, 18, 11)  PortDimensions=[4]  SampleTime=1e-08
  id_ref : Inport  Port=2  OutDataTypeStr=fixdt(1, 18, 11)  PortDimensions=1  SampleTime=1e-08
  iq_ref : Inport  Port=3  OutDataTypeStr=fixdt(1, 18, 11)  PortDimensions=1  SampleTime=1e-08
  ix_ref : Inport  Port=4  OutDataTypeStr=fixdt(1, 18, 11)  PortDimensions=1  SampleTime=1e-08
  iy_ref : Inport  Port=5  OutDataTypeStr=fixdt(1, 18, 11)  PortDimensions=1  SampleTime=1e-08
  Prediction_2_0_wire : hdlmdlgenlib/Buffer
      settings: SourceProductBaseCode=SL
  Prediction_2_1_wire : hdlmdlgenlib/Buffer
      settings: SourceProductBaseCode=SL
  Prediction_2_2_wire : hdlmdlgenlib/Buffer
      settings: SourceProductBaseCode=SL
  Prediction_2_3_wire : hdlmdlgenlib/Buffer
      settings: SourceProductBaseCode=SL
  Product{1..4} (4 alike) : Product  Inputs=**  OutDataTypeStr=fixdt(1, 20, 11)  SampleTime=1e-08
  Subtract{4..7} (4 alike) : Sum  Inputs=+-  AccumDataTypeStr=fixdt(1, 19, 11)  OutDataTypeStr=fixdt(1, 20, 11)  SampleTime=1e-08
  Sum of Elements_stage2 : Sum  AccumDataTypeStr=fixdt(1, 22, 11)  OutDataTypeStr=fixdt(1, 21, 11)  SampleTime=1e-08
  Sum of Elements_stage3 : Sum  AccumDataTypeStr=fixdt(1, 22, 11)  OutDataTypeStr=fixdt(1, 22, 11)  SampleTime=1e-08
  Sum of Elements_stage4 : Sum  AccumDataTypeStr=fixdt(1, 22, 11)  OutDataTypeStr=fixdt(1, 20, 11)  SampleTime=1e-08
  t : Demux
  J2 : Outport  SampleTime=1e-08
  wires:
  Prediction_2/1 -> t/1
  id_ref/1 -> Subtract4/1
  iq_ref/1 -> Subtract5/1
  ix_ref/1 -> Subtract6/1
  iy_ref/1 -> Subtract7/1
  Prediction_2_0_wire/1 -> Subtract4/2
  Prediction_2_1_wire/1 -> Subtract5/2
  Prediction_2_2_wire/1 -> Subtract6/2
  Prediction_2_3_wire/1 -> Subtract7/2
  Product1/1 -> Sum of Elements_stage2/2
  Product2/1 -> Sum of Elements_stage3/2
  Product3/1 -> Sum of Elements_stage2/1
  Product4/1 -> Sum of Elements_stage4/2
  Subtract4/1 -> Product3/2, Product3/1
  Subtract5/1 -> Product1/2, Product1/1
  Subtract6/1 -> Product2/2, Product2/1
  Subtract7/1 -> Product4/2, Product4/1
  Sum of Elements_stage4/1 -> J2/1
  t/1 -> Prediction_2_0_wire/1
  t/2 -> Prediction_2_1_wire/1
  t/3 -> Prediction_2_2_wire/1
  t/4 -> Prediction_2_3_wire/1
  Sum of Elements_stage2/1 -> Sum of Elements_stage3/1
  Sum of Elements_stage3/1 -> Sum of Elements_stage4/1

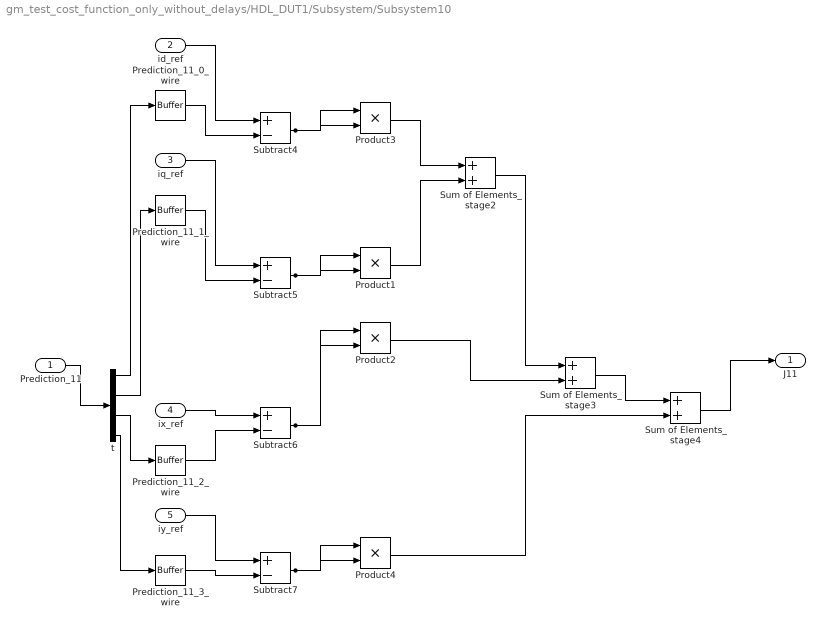
== system gm_test_cost_function_only_without_delays/HDL_DUT1/Subsystem/Subsystem10 ==
  Prediction_11 : Inport  OutDataTypeStr=fixdt(1, 18, 11)  PortDimensions=[4]  SampleTime=1e-08
  id_ref : Inport  Port=2  OutDataTypeStr=fixdt(1, 18, 11)  PortDimensions=1  SampleTime=1e-08
  iq_ref : Inport  Port=3  OutDataTypeStr=fixdt(1, 18, 11)  PortDimensions=1  SampleTime=1e-08
  ix_ref : Inport  Port=4  OutDataTypeStr=fixdt(1, 18, 11)  PortDimensions=1  SampleTime=1e-08
  iy_ref : Inport  Port=5  OutDataTypeStr=fixdt(1, 18, 11)  PortDimensions=1  SampleTime=1e-08
  Prediction_11_0_wire : hdlmdlgenlib/Buffer
      settings: SourceProductBaseCode=SL
  Prediction_11_1_wire : hdlmdlgenlib/Buffer
      settings: SourceProductBaseCode=SL
  Prediction_11_2_wire : hdlmdlgenlib/Buffer
      settings: SourceProductBaseCode=SL
  Prediction_11_3_wire : hdlmdlgenlib/Buffer
      settings: SourceProductBaseCode=SL
  Product{1..4} (4 alike) : Product  Inputs=**  OutDataTypeStr=fixdt(1, 20, 11)  SampleTime=1e-08
  Subtract{4..7} (4 alike) : Sum  Inputs=+-  AccumDataTypeStr=fixdt(1, 19, 11)  OutDataTypeStr=fixdt(1, 20, 11)  SampleTime=1e-08
  Sum of Elements_stage2 : Sum  AccumDataTypeStr=fixdt(1, 22, 11)  OutDataTypeStr=fixdt(1, 21, 11)  SampleTime=1e-08
  Sum of Elements_stage3 : Sum  AccumDataTypeStr=fixdt(1, 22, 11)  OutDataTypeStr=fixdt(1, 22, 11)  SampleTime=1e-08
  Sum of Elements_stage4 : Sum  AccumDataTypeStr=fixdt(1, 22, 11)  OutDataTypeStr=fixdt(1, 20, 11)  SampleTime=1e-08
  t : Demux
  J11 : Outport  SampleTime=1e-08
  wires:
  Prediction_11/1 -> t/1
  id_ref/1 -> Subtract4/1
  iq_ref/1 -> Subtract5/1
  ix_ref/1 -> Subtract6/1
  iy_ref/1 -> Subtract7/1
  Prediction_11_0_wire/1 -> Subtract4/2
  Prediction_11_1_wire/1 -> Subtract5/2
  Prediction_11_2_wire/1 -> Subtract6/2
  Prediction_11_3_wire/1 -> Subtract7/2
  Product1/1 -> Sum of Elements_stage2/2
  Product2/1 -> Sum of Elements_stage3/2
  Product3/1 -> Sum of Elements_stage2/1
  Product4/1 -> Sum of Elements_stage4/2
  Subtract4/1 -> Product3/2, Product3/1
  Subtract5/1 -> Product1/2, Product1/1
  Subtract6/1 -> Product2/2, Product2/1
  Subtract7/1 -> Product4/2, Product4/1
  Sum of Elements_stage4/1 -> J11/1
  t/1 -> Prediction_11_0_wire/1
  t/2 -> Prediction_11_1_wire/1
  t/3 -> Prediction_11_2_wire/1
  t/4 -> Prediction_11_3_wire/1
  Sum of Elements_stage2/1 -> Sum of Elements_stage3/1
  Sum of Elements_stage3/1 -> Sum of Elements_stage4/1

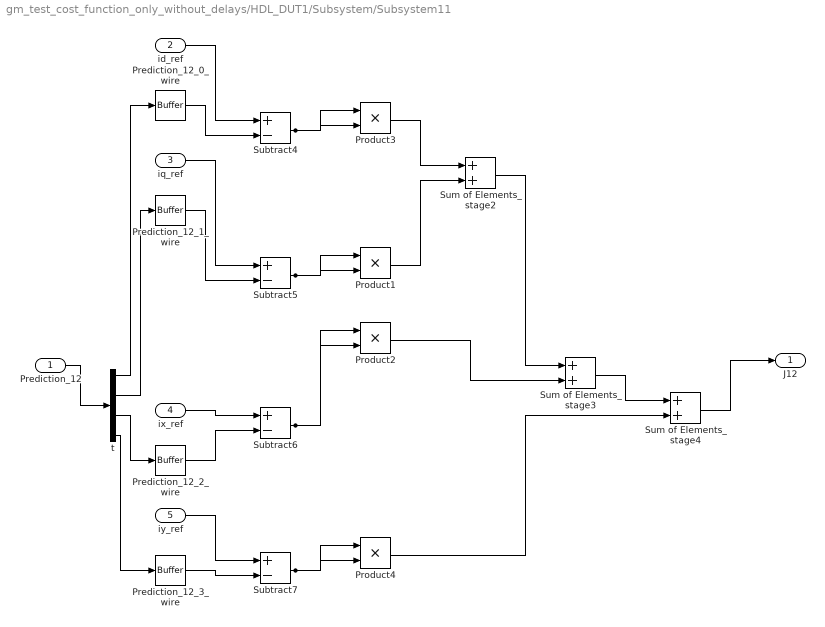
== system gm_test_cost_function_only_without_delays/HDL_DUT1/Subsystem/Subsystem11 ==
  Prediction_12 : Inport  OutDataTypeStr=fixdt(1, 18, 11)  PortDimensions=[4]  SampleTime=1e-08
  id_ref : Inport  Port=2  OutDataTypeStr=fixdt(1, 18, 11)  PortDimensions=1  SampleTime=1e-08
  iq_ref : Inport  Port=3  OutDataTypeStr=fixdt(1, 18, 11)  PortDimensions=1  SampleTime=1e-08
  ix_ref : Inport  Port=4  OutDataTypeStr=fixdt(1, 18, 11)  PortDimensions=1  SampleTime=1e-08
  iy_ref : Inport  Port=5  OutDataTypeStr=fixdt(1, 18, 11)  PortDimensions=1  SampleTime=1e-08
  Prediction_12_0_wire : hdlmdlgenlib/Buffer
      settings: SourceProductBaseCode=SL
  Prediction_12_1_wire : hdlmdlgenlib/Buffer
      settings: SourceProductBaseCode=SL
  Prediction_12_2_wire : hdlmdlgenlib/Buffer
      settings: SourceProductBaseCode=SL
  Prediction_12_3_wire : hdlmdlgenlib/Buffer
      settings: SourceProductBaseCode=SL
  Product{1..4} (4 alike) : Product  Inputs=**  OutDataTypeStr=fixdt(1, 20, 11)  SampleTime=1e-08
  Subtract{4..7} (4 alike) : Sum  Inputs=+-  AccumDataTypeStr=fixdt(1, 19, 11)  OutDataTypeStr=fixdt(1, 20, 11)  SampleTime=1e-08
  Sum of Elements_stage2 : Sum  AccumDataTypeStr=fixdt(1, 22, 11)  OutDataTypeStr=fixdt(1, 21, 11)  SampleTime=1e-08
  Sum of Elements_stage3 : Sum  AccumDataTypeStr=fixdt(1, 22, 11)  OutDataTypeStr=fixdt(1, 22, 11)  SampleTime=1e-08
  Sum of Elements_stage4 : Sum  AccumDataTypeStr=fixdt(1, 22, 11)  OutDataTypeStr=fixdt(1, 20, 11)  SampleTime=1e-08
  t : Demux
  J12 : Outport  SampleTime=1e-08
  wires:
  Prediction_12/1 -> t/1
  id_ref/1 -> Subtract4/1
  iq_ref/1 -> Subtract5/1
  ix_ref/1 -> Subtract6/1
  iy_ref/1 -> Subtract7/1
  Prediction_12_0_wire/1 -> Subtract4/2
  Prediction_12_1_wire/1 -> Subtract5/2
  Prediction_12_2_wire/1 -> Subtract6/2
  Prediction_12_3_wire/1 -> Subtract7/2
  Product1/1 -> Sum of Elements_stage2/2
  Product2/1 -> Sum of Elements_stage3/2
  Product3/1 -> Sum of Elements_stage2/1
  Product4/1 -> Sum of Elements_stage4/2
  Subtract4/1 -> Product3/2, Product3/1
  Subtract5/1 -> Product1/2, Product1/1
  Subtract6/1 -> Product2/2, Product2/1
  Subtract7/1 -> Product4/2, Product4/1
  Sum of Elements_stage4/1 -> J12/1
  t/1 -> Prediction_12_0_wire/1
  t/2 -> Prediction_12_1_wire/1
  t/3 -> Prediction_12_2_wire/1
  t/4 -> Prediction_12_3_wire/1
  Sum of Elements_stage2/1 -> Sum of Elements_stage3/1
  Sum of Elements_stage3/1 -> Sum of Elements_stage4/1

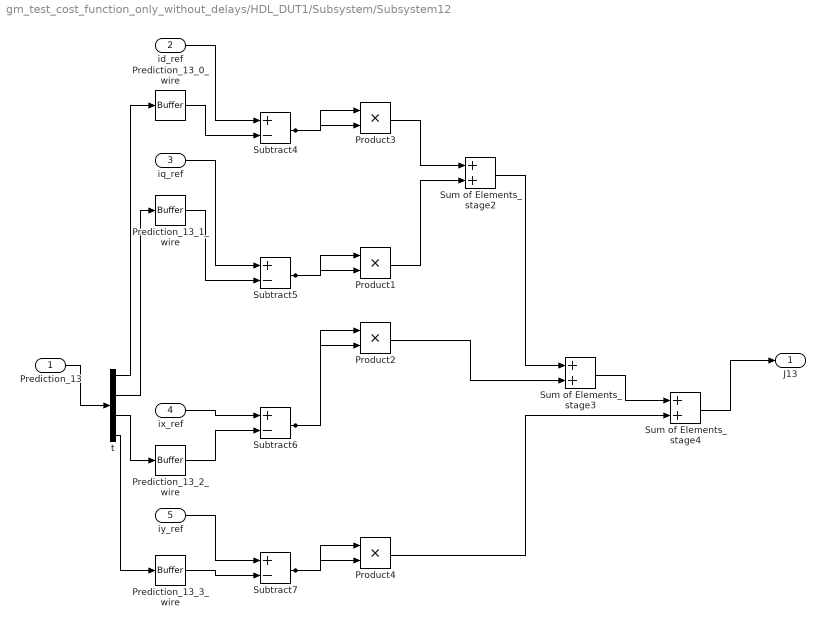
== system gm_test_cost_function_only_without_delays/HDL_DUT1/Subsystem/Subsystem12 ==
  Prediction_13 : Inport  OutDataTypeStr=fixdt(1, 18, 11)  PortDimensions=[4]  SampleTime=1e-08
  id_ref : Inport  Port=2  OutDataTypeStr=fixdt(1, 18, 11)  PortDimensions=1  SampleTime=1e-08
  iq_ref : Inport  Port=3  OutDataTypeStr=fixdt(1, 18, 11)  PortDimensions=1  SampleTime=1e-08
  ix_ref : Inport  Port=4  OutDataTypeStr=fixdt(1, 18, 11)  PortDimensions=1  SampleTime=1e-08
  iy_ref : Inport  Port=5  OutDataTypeStr=fixdt(1, 18, 11)  PortDimensions=1  SampleTime=1e-08
  Prediction_13_0_wire : hdlmdlgenlib/Buffer
      settings: SourceProductBaseCode=SL
  Prediction_13_1_wire : hdlmdlgenlib/Buffer
      settings: SourceProductBaseCode=SL
  Prediction_13_2_wire : hdlmdlgenlib/Buffer
      settings: SourceProductBaseCode=SL
  Prediction_13_3_wire : hdlmdlgenlib/Buffer
      settings: SourceProductBaseCode=SL
  Product{1..4} (4 alike) : Product  Inputs=**  OutDataTypeStr=fixdt(1, 20, 11)  SampleTime=1e-08
  Subtract{4..7} (4 alike) : Sum  Inputs=+-  AccumDataTypeStr=fixdt(1, 19, 11)  OutDataTypeStr=fixdt(1, 20, 11)  SampleTime=1e-08
  Sum of Elements_stage2 : Sum  AccumDataTypeStr=fixdt(1, 22, 11)  OutDataTypeStr=fixdt(1, 21, 11)  SampleTime=1e-08
  Sum of Elements_stage3 : Sum  AccumDataTypeStr=fixdt(1, 22, 11)  OutDataTypeStr=fixdt(1, 22, 11)  SampleTime=1e-08
  Sum of Elements_stage4 : Sum  AccumDataTypeStr=fixdt(1, 22, 11)  OutDataTypeStr=fixdt(1, 20, 11)  SampleTime=1e-08
  t : Demux
  J13 : Outport  SampleTime=1e-08
  wires:
  Prediction_13/1 -> t/1
  id_ref/1 -> Subtract4/1
  iq_ref/1 -> Subtract5/1
  ix_ref/1 -> Subtract6/1
  iy_ref/1 -> Subtract7/1
  Prediction_13_0_wire/1 -> Subtract4/2
  Prediction_13_1_wire/1 -> Subtract5/2
  Prediction_13_2_wire/1 -> Subtract6/2
  Prediction_13_3_wire/1 -> Subtract7/2
  Product1/1 -> Sum of Elements_stage2/2
  Product2/1 -> Sum of Elements_stage3/2
  Product3/1 -> Sum of Elements_stage2/1
  Product4/1 -> Sum of Elements_stage4/2
  Subtract4/1 -> Product3/2, Product3/1
  Subtract5/1 -> Product1/2, Product1/1
  Subtract6/1 -> Product2/2, Product2/1
  Subtract7/1 -> Product4/2, Product4/1
  Sum of Elements_stage4/1 -> J13/1
  t/1 -> Prediction_13_0_wire/1
  t/2 -> Prediction_13_1_wire/1
  t/3 -> Prediction_13_2_wire/1
  t/4 -> Prediction_13_3_wire/1
  Sum of Elements_stage2/1 -> Sum of Elements_stage3/1
  Sum of Elements_stage3/1 -> Sum of Elements_stage4/1

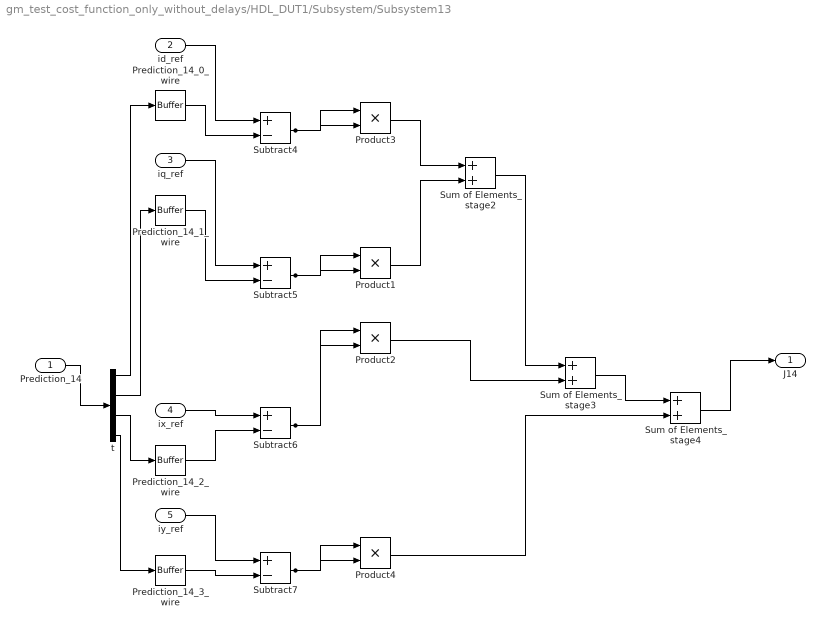
== system gm_test_cost_function_only_without_delays/HDL_DUT1/Subsystem/Subsystem13 ==
  Prediction_14 : Inport  OutDataTypeStr=fixdt(1, 18, 11)  PortDimensions=[4]  SampleTime=1e-08
  id_ref : Inport  Port=2  OutDataTypeStr=fixdt(1, 18, 11)  PortDimensions=1  SampleTime=1e-08
  iq_ref : Inport  Port=3  OutDataTypeStr=fixdt(1, 18, 11)  PortDimensions=1  SampleTime=1e-08
  ix_ref : Inport  Port=4  OutDataTypeStr=fixdt(1, 18, 11)  PortDimensions=1  SampleTime=1e-08
  iy_ref : Inport  Port=5  OutDataTypeStr=fixdt(1, 18, 11)  PortDimensions=1  SampleTime=1e-08
  Prediction_14_0_wire : hdlmdlgenlib/Buffer
      settings: SourceProductBaseCode=SL
  Prediction_14_1_wire : hdlmdlgenlib/Buffer
      settings: SourceProductBaseCode=SL
  Prediction_14_2_wire : hdlmdlgenlib/Buffer
      settings: SourceProductBaseCode=SL
  Prediction_14_3_wire : hdlmdlgenlib/Buffer
      settings: SourceProductBaseCode=SL
  Product{1..4} (4 alike) : Product  Inputs=**  OutDataTypeStr=fixdt(1, 20, 11)  SampleTime=1e-08
  Subtract{4..7} (4 alike) : Sum  Inputs=+-  AccumDataTypeStr=fixdt(1, 19, 11)  OutDataTypeStr=fixdt(1, 20, 11)  SampleTime=1e-08
  Sum of Elements_stage2 : Sum  AccumDataTypeStr=fixdt(1, 22, 11)  OutDataTypeStr=fixdt(1, 21, 11)  SampleTime=1e-08
  Sum of Elements_stage3 : Sum  AccumDataTypeStr=fixdt(1, 22, 11)  OutDataTypeStr=fixdt(1, 22, 11)  SampleTime=1e-08
  Sum of Elements_stage4 : Sum  AccumDataTypeStr=fixdt(1, 22, 11)  OutDataTypeStr=fixdt(1, 20, 11)  SampleTime=1e-08
  t : Demux
  J14 : Outport  SampleTime=1e-08
  wires:
  Prediction_14/1 -> t/1
  id_ref/1 -> Subtract4/1
  iq_ref/1 -> Subtract5/1
  ix_ref/1 -> Subtract6/1
  iy_ref/1 -> Subtract7/1
  Prediction_14_0_wire/1 -> Subtract4/2
  Prediction_14_1_wire/1 -> Subtract5/2
  Prediction_14_2_wire/1 -> Subtract6/2
  Prediction_14_3_wire/1 -> Subtract7/2
  Product1/1 -> Sum of Elements_stage2/2
  Product2/1 -> Sum of Elements_stage3/2
  Product3/1 -> Sum of Elements_stage2/1
  Product4/1 -> Sum of Elements_stage4/2
  Subtract4/1 -> Product3/2, Product3/1
  Subtract5/1 -> Product1/2, Product1/1
  Subtract6/1 -> Product2/2, Product2/1
  Subtract7/1 -> Product4/2, Product4/1
  Sum of Elements_stage4/1 -> J14/1
  t/1 -> Prediction_14_0_wire/1
  t/2 -> Prediction_14_1_wire/1
  t/3 -> Prediction_14_2_wire/1
  t/4 -> Prediction_14_3_wire/1
  Sum of Elements_stage2/1 -> Sum of Elements_stage3/1
  Sum of Elements_stage3/1 -> Sum of Elements_stage4/1

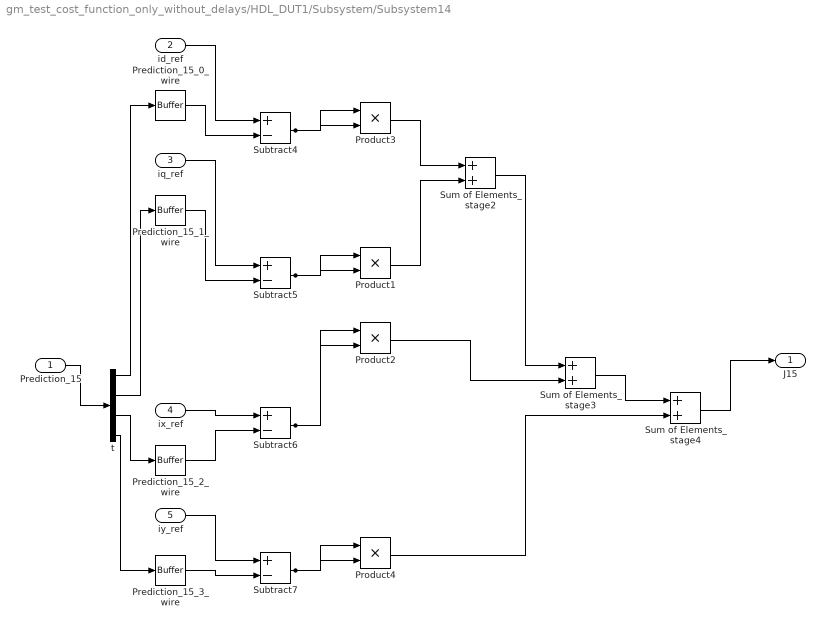
== system gm_test_cost_function_only_without_delays/HDL_DUT1/Subsystem/Subsystem14 ==
  Prediction_15 : Inport  OutDataTypeStr=fixdt(1, 18, 11)  PortDimensions=[4]  SampleTime=1e-08
  id_ref : Inport  Port=2  OutDataTypeStr=fixdt(1, 18, 11)  PortDimensions=1  SampleTime=1e-08
  iq_ref : Inport  Port=3  OutDataTypeStr=fixdt(1, 18, 11)  PortDimensions=1  SampleTime=1e-08
  ix_ref : Inport  Port=4  OutDataTypeStr=fixdt(1, 18, 11)  PortDimensions=1  SampleTime=1e-08
  iy_ref : Inport  Port=5  OutDataTypeStr=fixdt(1, 18, 11)  PortDimensions=1  SampleTime=1e-08
  Prediction_15_0_wire : hdlmdlgenlib/Buffer
      settings: SourceProductBaseCode=SL
  Prediction_15_1_wire : hdlmdlgenlib/Buffer
      settings: SourceProductBaseCode=SL
  Prediction_15_2_wire : hdlmdlgenlib/Buffer
      settings: SourceProductBaseCode=SL
  Prediction_15_3_wire : hdlmdlgenlib/Buffer
      settings: SourceProductBaseCode=SL
  Product{1..4} (4 alike) : Product  Inputs=**  OutDataTypeStr=fixdt(1, 20, 11)  SampleTime=1e-08
  Subtract{4..7} (4 alike) : Sum  Inputs=+-  AccumDataTypeStr=fixdt(1, 19, 11)  OutDataTypeStr=fixdt(1, 20, 11)  SampleTime=1e-08
  Sum of Elements_stage2 : Sum  AccumDataTypeStr=fixdt(1, 22, 11)  OutDataTypeStr=fixdt(1, 21, 11)  SampleTime=1e-08
  Sum of Elements_stage3 : Sum  AccumDataTypeStr=fixdt(1, 22, 11)  OutDataTypeStr=fixdt(1, 22, 11)  SampleTime=1e-08
  Sum of Elements_stage4 : Sum  AccumDataTypeStr=fixdt(1, 22, 11)  OutDataTypeStr=fixdt(1, 20, 11)  SampleTime=1e-08
  t : Demux
  J15 : Outport  SampleTime=1e-08
  wires:
  Prediction_15/1 -> t/1
  id_ref/1 -> Subtract4/1
  iq_ref/1 -> Subtract5/1
  ix_ref/1 -> Subtract6/1
  iy_ref/1 -> Subtract7/1
  Prediction_15_0_wire/1 -> Subtract4/2
  Prediction_15_1_wire/1 -> Subtract5/2
  Prediction_15_2_wire/1 -> Subtract6/2
  Prediction_15_3_wire/1 -> Subtract7/2
  Product1/1 -> Sum of Elements_stage2/2
  Product2/1 -> Sum of Elements_stage3/2
  Product3/1 -> Sum of Elements_stage2/1
  Product4/1 -> Sum of Elements_stage4/2
  Subtract4/1 -> Product3/2, Product3/1
  Subtract5/1 -> Product1/2, Product1/1
  Subtract6/1 -> Product2/2, Product2/1
  Subtract7/1 -> Product4/2, Product4/1
  Sum of Elements_stage4/1 -> J15/1
  t/1 -> Prediction_15_0_wire/1
  t/2 -> Prediction_15_1_wire/1
  t/3 -> Prediction_15_2_wire/1
  t/4 -> Prediction_15_3_wire/1
  Sum of Elements_stage2/1 -> Sum of Elements_stage3/1
  Sum of Elements_stage3/1 -> Sum of Elements_stage4/1

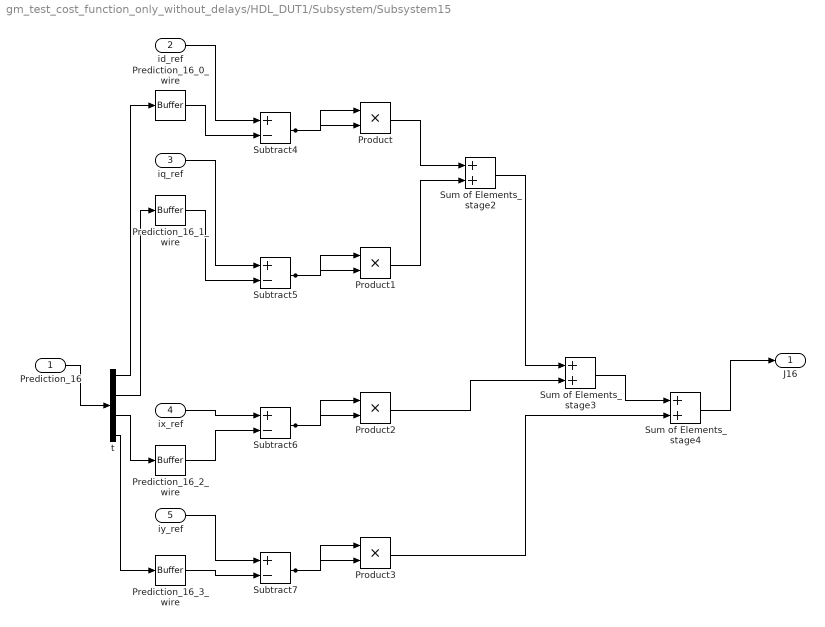
== system gm_test_cost_function_only_without_delays/HDL_DUT1/Subsystem/Subsystem15 ==
  Prediction_16 : Inport  OutDataTypeStr=fixdt(1, 18, 11)  PortDimensions=[4]  SampleTime=1e-08
  id_ref : Inport  Port=2  OutDataTypeStr=fixdt(1, 18, 11)  PortDimensions=1  SampleTime=1e-08
  iq_ref : Inport  Port=3  OutDataTypeStr=fixdt(1, 18, 11)  PortDimensions=1  SampleTime=1e-08
  ix_ref : Inport  Port=4  OutDataTypeStr=fixdt(1, 18, 11)  PortDimensions=1  SampleTime=1e-08
  iy_ref : Inport  Port=5  OutDataTypeStr=fixdt(1, 18, 11)  PortDimensions=1  SampleTime=1e-08
  Prediction_16_0_wire : hdlmdlgenlib/Buffer
      settings: SourceProductBaseCode=SL
  Prediction_16_1_wire : hdlmdlgenlib/Buffer
      settings: SourceProductBaseCode=SL
  Prediction_16_2_wire : hdlmdlgenlib/Buffer
      settings: SourceProductBaseCode=SL
  Prediction_16_3_wire : hdlmdlgenlib/Buffer
      settings: SourceProductBaseCode=SL
  Product{,1..3} (4 alike) : Product  Inputs=**  OutDataTypeStr=fixdt(1, 20, 11)  SampleTime=1e-08
  Subtract{4..7} (4 alike) : Sum  Inputs=+-  AccumDataTypeStr=fixdt(1, 19, 11)  OutDataTypeStr=fixdt(1, 20, 11)  SampleTime=1e-08
  Sum of Elements_stage2 : Sum  AccumDataTypeStr=fixdt(1, 22, 11)  OutDataTypeStr=fixdt(1, 21, 11)  SampleTime=1e-08
  Sum of Elements_stage3 : Sum  AccumDataTypeStr=fixdt(1, 22, 11)  OutDataTypeStr=fixdt(1, 22, 11)  SampleTime=1e-08
  Sum of Elements_stage4 : Sum  AccumDataTypeStr=fixdt(1, 22, 11)  OutDataTypeStr=fixdt(1, 20, 11)  SampleTime=1e-08
  t : Demux
  J16 : Outport  SampleTime=1e-08
  wires:
  Prediction_16/1 -> t/1
  id_ref/1 -> Subtract4/1
  iq_ref/1 -> Subtract5/1
  ix_ref/1 -> Subtract6/1
  iy_ref/1 -> Subtract7/1
  Prediction_16_0_wire/1 -> Subtract4/2
  Prediction_16_1_wire/1 -> Subtract5/2
  Prediction_16_2_wire/1 -> Subtract6/2
  Prediction_16_3_wire/1 -> Subtract7/2
  Product/1 -> Sum of Elements_stage2/1
  Product1/1 -> Sum of Elements_stage2/2
  Product2/1 -> Sum of Elements_stage3/2
  Product3/1 -> Sum of Elements_stage4/2
  Subtract4/1 -> Product/2, Product/1
  Subtract5/1 -> Product1/2, Product1/1
  Subtract6/1 -> Product2/2, Product2/1
  Subtract7/1 -> Product3/2, Product3/1
  Sum of Elements_stage4/1 -> J16/1
  t/1 -> Prediction_16_0_wire/1
  t/2 -> Prediction_16_1_wire/1
  t/3 -> Prediction_16_2_wire/1
  t/4 -> Prediction_16_3_wire/1
  Sum of Elements_stage2/1 -> Sum of Elements_stage3/1
  Sum of Elements_stage3/1 -> Sum of Elements_stage4/1

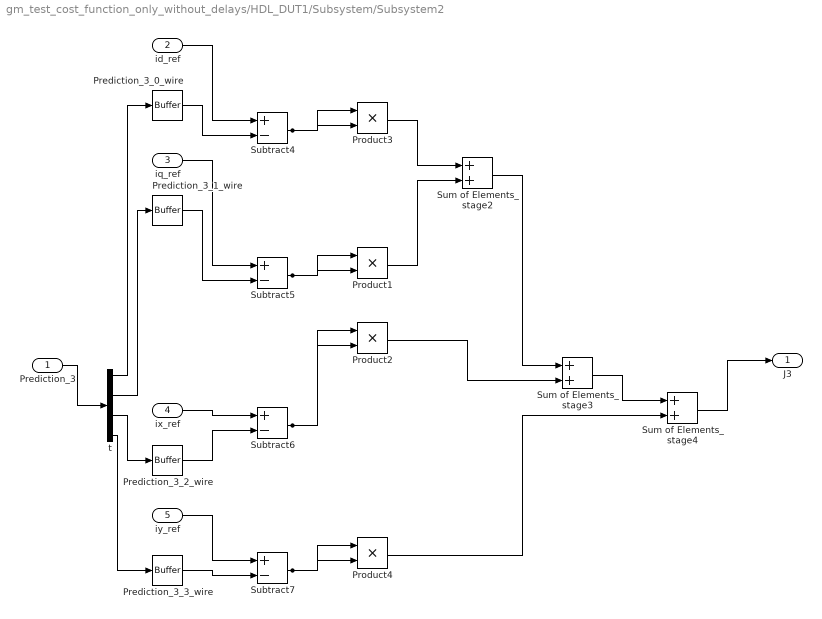
== system gm_test_cost_function_only_without_delays/HDL_DUT1/Subsystem/Subsystem2 ==
  Prediction_3 : Inport  OutDataTypeStr=fixdt(1, 18, 11)  PortDimensions=[4]  SampleTime=1e-08
  id_ref : Inport  Port=2  OutDataTypeStr=fixdt(1, 18, 11)  PortDimensions=1  SampleTime=1e-08
  iq_ref : Inport  Port=3  OutDataTypeStr=fixdt(1, 18, 11)  PortDimensions=1  SampleTime=1e-08
  ix_ref : Inport  Port=4  OutDataTypeStr=fixdt(1, 18, 11)  PortDimensions=1  SampleTime=1e-08
  iy_ref : Inport  Port=5  OutDataTypeStr=fixdt(1, 18, 11)  PortDimensions=1  SampleTime=1e-08
  Prediction_3_0_wire : hdlmdlgenlib/Buffer
      settings: SourceProductBaseCode=SL
  Prediction_3_1_wire : hdlmdlgenlib/Buffer
      settings: SourceProductBaseCode=SL
  Prediction_3_2_wire : hdlmdlgenlib/Buffer
      settings: SourceProductBaseCode=SL
  Prediction_3_3_wire : hdlmdlgenlib/Buffer
      settings: SourceProductBaseCode=SL
  Product{1..4} (4 alike) : Product  Inputs=**  OutDataTypeStr=fixdt(1, 20, 11)  SampleTime=1e-08
  Subtract{4..7} (4 alike) : Sum  Inputs=+-  AccumDataTypeStr=fixdt(1, 19, 11)  OutDataTypeStr=fixdt(1, 20, 11)  SampleTime=1e-08
  Sum of Elements_stage2 : Sum  AccumDataTypeStr=fixdt(1, 22, 11)  OutDataTypeStr=fixdt(1, 21, 11)  SampleTime=1e-08
  Sum of Elements_stage3 : Sum  AccumDataTypeStr=fixdt(1, 22, 11)  OutDataTypeStr=fixdt(1, 22, 11)  SampleTime=1e-08
  Sum of Elements_stage4 : Sum  AccumDataTypeStr=fixdt(1, 22, 11)  OutDataTypeStr=fixdt(1, 20, 11)  SampleTime=1e-08
  t : Demux
  J3 : Outport  SampleTime=1e-08
  wires:
  Prediction_3/1 -> t/1
  id_ref/1 -> Subtract4/1
  iq_ref/1 -> Subtract5/1
  ix_ref/1 -> Subtract6/1
  iy_ref/1 -> Subtract7/1
  Prediction_3_0_wire/1 -> Subtract4/2
  Prediction_3_1_wire/1 -> Subtract5/2
  Prediction_3_2_wire/1 -> Subtract6/2
  Prediction_3_3_wire/1 -> Subtract7/2
  Product1/1 -> Sum of Elements_stage2/2
  Product2/1 -> Sum of Elements_stage3/2
  Product3/1 -> Sum of Elements_stage2/1
  Product4/1 -> Sum of Elements_stage4/2
  Subtract4/1 -> Product3/2, Product3/1
  Subtract5/1 -> Product1/2, Product1/1
  Subtract6/1 -> Product2/2, Product2/1
  Subtract7/1 -> Product4/2, Product4/1
  Sum of Elements_stage4/1 -> J3/1
  t/1 -> Prediction_3_0_wire/1
  t/2 -> Prediction_3_1_wire/1
  t/3 -> Prediction_3_2_wire/1
  t/4 -> Prediction_3_3_wire/1
  Sum of Elements_stage2/1 -> Sum of Elements_stage3/1
  Sum of Elements_stage3/1 -> Sum of Elements_stage4/1

== system gm_test_cost_function_only_without_delays/HDL_DUT1/Subsystem/Subsystem3 ==
  Prediction_4 : Inport  OutDataTypeStr=fixdt(1, 18, 11)  PortDimensions=[4]  SampleTime=1e-08
  id_ref : Inport  Port=2  OutDataTypeStr=fixdt(1, 18, 11)  PortDimensions=1  SampleTime=1e-08
  iq_ref : Inport  Port=3  OutDataTypeStr=fixdt(1, 18, 11)  PortDimensions=1  SampleTime=1e-08
  ix_ref : Inport  Port=4  OutDataTypeStr=fixdt(1, 18, 11)  PortDimensions=1  SampleTime=1e-08
  iy_ref : Inport  Port=5  OutDataTypeStr=fixdt(1, 18, 11)  PortDimensions=1  SampleTime=1e-08
  Prediction_4_0_wire : hdlmdlgenlib/Buffer
      settings: SourceProductBaseCode=SL
  Prediction_4_1_wire : hdlmdlgenlib/Buffer
      settings: SourceProductBaseCode=SL
  Prediction_4_2_wire : hdlmdlgenlib/Buffer
      settings: SourceProductBaseCode=SL
  Prediction_4_3_wire : hdlmdlgenlib/Buffer
      settings: SourceProductBaseCode=SL
  Product{1..4} (4 alike) : Product  Inputs=**  OutDataTypeStr=fixdt(1, 20, 11)  SampleTime=1e-08
  Subtract{4..7} (4 alike) : Sum  Inputs=+-  AccumDataTypeStr=fixdt(1, 19, 11)  OutDataTypeStr=fixdt(1, 20, 11)  SampleTime=1e-08
  Sum of Elements_stage2 : Sum  AccumDataTypeStr=fixdt(1, 22, 11)  OutDataTypeStr=fixdt(1, 21, 11)  SampleTime=1e-08
  Sum of Elements_stage3 : Sum  AccumDataTypeStr=fixdt(1, 22, 11)  OutDataTypeStr=fixdt(1, 22, 11)  SampleTime=1e-08
  Sum of Elements_stage4 : Sum  AccumDataTypeStr=fixdt(1, 22, 11)  OutDataTypeStr=fixdt(1, 20, 11)  SampleTime=1e-08
  t : Demux
  J4 : Outport  SampleTime=1e-08
  wires:
  Prediction_4/1 -> t/1
  id_ref/1 -> Subtract4/1
  iq_ref/1 -> Subtract5/1
  ix_ref/1 -> Subtract6/1
  iy_ref/1 -> Subtract7/1
  Prediction_4_0_wire/1 -> Subtract4/2
  Prediction_4_1_wire/1 -> Subtract5/2
  Prediction_4_2_wire/1 -> Subtract6/2
  Prediction_4_3_wire/1 -> Subtract7/2
  Product1/1 -> Sum of Elements_stage2/2
  Product2/1 -> Sum of Elements_stage3/2
  Product3/1 -> Sum of Elements_stage2/1
  Product4/1 -> Sum of Elements_stage4/2
  Subtract4/1 -> Product3/2, Product3/1
  Subtract5/1 -> Product1/2, Product1/1
  Subtract6/1 -> Product2/2, Product2/1
  Subtract7/1 -> Product4/2, Product4/1
  Sum of Elements_stage4/1 -> J4/1
  t/1 -> Prediction_4_0_wire/1
  t/2 -> Prediction_4_1_wire/1
  t/3 -> Prediction_4_2_wire/1
  t/4 -> Prediction_4_3_wire/1
  Sum of Elements_stage2/1 -> Sum of Elements_stage3/1
  Sum of Elements_stage3/1 -> Sum of Elements_stage4/1
